simulink model "darkquad17"  (R2012b)
settings: Solver=VariableStepDiscrete  SolverMode=SingleTasking  StartTime=0.0  StopTime=10000  RelTol=1e-3
libraries: xbsIndex_r4 x6460, casper_library_misc x74, casper_library_flow_control x8, xps_library x7
(part 29 of 59)

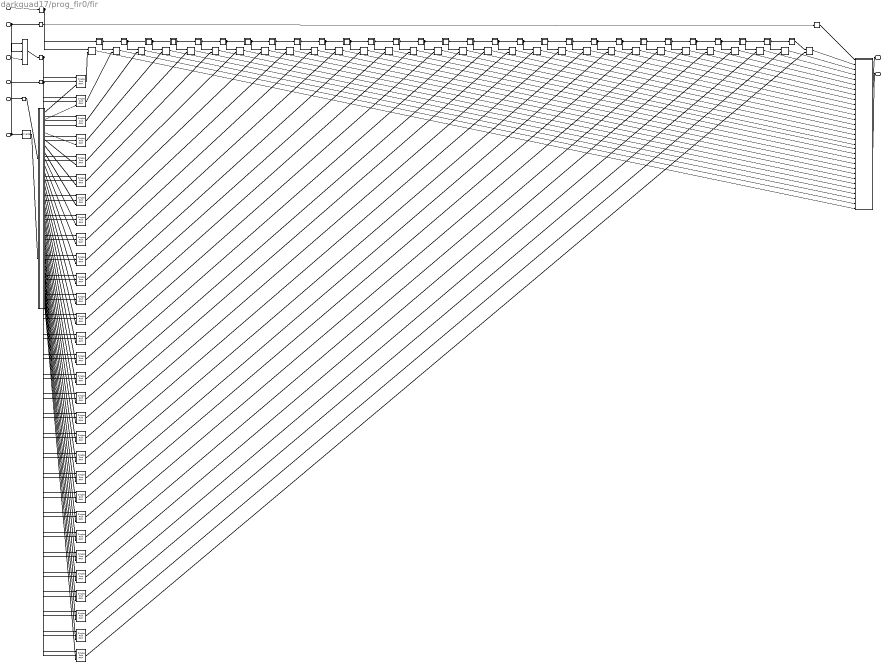
== system darkquad17/prog_fir0/fir ==
  data_in : Inport
  ch_in : Inport  Port=2
  write_coeff : Inport  Port=3
  coeff_to_write : Inport  Port=4
  tap_to_write : Inport  Port=5
  ch_to_write : Inport  Port=6
  Mult{1..30} (30 alike) : xbsIndex_r4/Mult  precision=Full  arith_type="Signed  (2's comp)"  n_bits=16  bin_pt=14  quantization=Truncate  overflow=Wrap  en=off  latency=4  dbl_ovrd=off  use_behavioral_HDL=off  opt=Speed  use_embedded=on  optimum_pipeline=on  pipeline=on  use_rpm=on  placement_style=Triangular  block_type=mult
  bram{1..30} (30 alike) : xbsIndex_r4/Single Port RAM  depth=256  initVector=0  distributed_mem=Block RAM  write_mode=No Read On Write  rst=off  init_reg=0  en=off  latency=3  dbl_ovrd=off  optimize=Area  block_type=spram
  ch_dly : xbsIndex_r4/Delay  rst=off  infoeditControl=Selection of Reset will increase slice count due to use of real FFs and instead of SRLs  en=off  latency=2  dbl_ovrd=off  reg_retiming=off  block_type=delay
  ch_mux : xbsIndex_r4/Mux  inputs=2  en=off  latency=1  precision=Full  arith_type=Unsigned  n_bits=16  bin_pt=14  quantization=Truncate  overflow=Wrap  dbl_ovrd=off  block_type=mux
  coeff_in_dly : xbsIndex_r4/Delay  rst=off  infoeditControl=Selection of Reset will increase slice count due to use of real FFs and instead of SRLs  en=off  latency=3  dbl_ovrd=off  reg_retiming=off  block_type=delay
  data_dly : xbsIndex_r4/Delay  rst=off  infoeditControl=Selection of Reset will increase slice count due to use of real FFs and instead of SRLs  en=off  latency=6  dbl_ovrd=off  reg_retiming=off  block_type=delay
  delay1 : Subsystem  mask(delay_bram){DelayLen=256, bram_latency=2, implementation=Fabric, async=off}
      mask prompts: DelayLen "Delay By:"; bram_latency "BRAM Latency"; implementation "Implement using"; async "asynchronous operation"
      mask help: A delay block that uses BRAM for its storage.
      mask init:
      | delay_bram_impl_init(gcb, ...
      |     'DelayLen', DelayLen, ...
      |     'bram_latency', bram_latency, ...
      |     'implementation', implementation, ...
      |     'async', async);
      mask Help: eval('xlWeb(''http://casper.berkeley.edu/wiki/Delay_bram'')')
      mask TypeOptions implementation: Behavioral HDL | Fabric | DSP48
      mask Display:
      | str=sprintf('z^{-%d}',DelayLen);
      | color('black');disp(str,'texmode','on');
  delay10 : Subsystem  mask(delay_bram){DelayLen=256, bram_latency=2, implementation=Fabric, async=off}
      mask prompts: DelayLen "Delay By:"; bram_latency "BRAM Latency"; implementation "Implement using"; async "asynchronous operation"
      mask help: A delay block that uses BRAM for its storage.
      mask init:
      | delay_bram_impl_init(gcb, ...
      |     'DelayLen', DelayLen, ...
      |     'bram_latency', bram_latency, ...
      |     'implementation', implementation, ...
      |     'async', async);
      mask Help: eval('xlWeb(''http://casper.berkeley.edu/wiki/Delay_bram'')')
      mask TypeOptions implementation: Behavioral HDL | Fabric | DSP48
      mask Display:
      | str=sprintf('z^{-%d}',DelayLen);
      | color('black');disp(str,'texmode','on');
  delay11 : Subsystem  mask(delay_bram){DelayLen=256, bram_latency=2, implementation=Fabric, async=off}
      mask prompts: DelayLen "Delay By:"; bram_latency "BRAM Latency"; implementation "Implement using"; async "asynchronous operation"
      mask help: A delay block that uses BRAM for its storage.
      mask init:
      | delay_bram_impl_init(gcb, ...
      |     'DelayLen', DelayLen, ...
      |     'bram_latency', bram_latency, ...
      |     'implementation', implementation, ...
      |     'async', async);
      mask Help: eval('xlWeb(''http://casper.berkeley.edu/wiki/Delay_bram'')')
      mask TypeOptions implementation: Behavioral HDL | Fabric | DSP48
      mask Display:
      | str=sprintf('z^{-%d}',DelayLen);
      | color('black');disp(str,'texmode','on');
  delay12 : Subsystem  mask(delay_bram){DelayLen=256, bram_latency=2, implementation=Fabric, async=off}
      mask prompts: DelayLen "Delay By:"; bram_latency "BRAM Latency"; implementation "Implement using"; async "asynchronous operation"
      mask help: A delay block that uses BRAM for its storage.
      mask init:
      | delay_bram_impl_init(gcb, ...
      |     'DelayLen', DelayLen, ...
      |     'bram_latency', bram_latency, ...
      |     'implementation', implementation, ...
      |     'async', async);
      mask Help: eval('xlWeb(''http://casper.berkeley.edu/wiki/Delay_bram'')')
      mask TypeOptions implementation: Behavioral HDL | Fabric | DSP48
      mask Display:
      | str=sprintf('z^{-%d}',DelayLen);
      | color('black');disp(str,'texmode','on');
  delay13 : Subsystem  mask(delay_bram){DelayLen=256, bram_latency=2, implementation=Fabric, async=off}
      mask prompts: DelayLen "Delay By:"; bram_latency "BRAM Latency"; implementation "Implement using"; async "asynchronous operation"
      mask help: A delay block that uses BRAM for its storage.
      mask init:
      | delay_bram_impl_init(gcb, ...
      |     'DelayLen', DelayLen, ...
      |     'bram_latency', bram_latency, ...
      |     'implementation', implementation, ...
      |     'async', async);
      mask Help: eval('xlWeb(''http://casper.berkeley.edu/wiki/Delay_bram'')')
      mask TypeOptions implementation: Behavioral HDL | Fabric | DSP48
      mask Display:
      | str=sprintf('z^{-%d}',DelayLen);
      | color('black');disp(str,'texmode','on');
  delay14 : Subsystem  mask(delay_bram){DelayLen=256, bram_latency=2, implementation=Fabric, async=off}
      mask prompts: DelayLen "Delay By:"; bram_latency "BRAM Latency"; implementation "Implement using"; async "asynchronous operation"
      mask help: A delay block that uses BRAM for its storage.
      mask init:
      | delay_bram_impl_init(gcb, ...
      |     'DelayLen', DelayLen, ...
      |     'bram_latency', bram_latency, ...
      |     'implementation', implementation, ...
      |     'async', async);
      mask Help: eval('xlWeb(''http://casper.berkeley.edu/wiki/Delay_bram'')')
      mask TypeOptions implementation: Behavioral HDL | Fabric | DSP48
      mask Display:
      | str=sprintf('z^{-%d}',DelayLen);
      | color('black');disp(str,'texmode','on');
  delay15 : Subsystem  mask(delay_bram){DelayLen=256, bram_latency=2, implementation=Fabric, async=off}
      mask prompts: DelayLen "Delay By:"; bram_latency "BRAM Latency"; implementation "Implement using"; async "asynchronous operation"
      mask help: A delay block that uses BRAM for its storage.
      mask init:
      | delay_bram_impl_init(gcb, ...
      |     'DelayLen', DelayLen, ...
      |     'bram_latency', bram_latency, ...
      |     'implementation', implementation, ...
      |     'async', async);
      mask Help: eval('xlWeb(''http://casper.berkeley.edu/wiki/Delay_bram'')')
      mask TypeOptions implementation: Behavioral HDL | Fabric | DSP48
      mask Display:
      | str=sprintf('z^{-%d}',DelayLen);
      | color('black');disp(str,'texmode','on');
  delay16 : Subsystem  mask(delay_bram){DelayLen=256, bram_latency=2, implementation=Fabric, async=off}
      mask prompts: DelayLen "Delay By:"; bram_latency "BRAM Latency"; implementation "Implement using"; async "asynchronous operation"
      mask help: A delay block that uses BRAM for its storage.
      mask init:
      | delay_bram_impl_init(gcb, ...
      |     'DelayLen', DelayLen, ...
      |     'bram_latency', bram_latency, ...
      |     'implementation', implementation, ...
      |     'async', async);
      mask Help: eval('xlWeb(''http://casper.berkeley.edu/wiki/Delay_bram'')')
      mask TypeOptions implementation: Behavioral HDL | Fabric | DSP48
      mask Display:
      | str=sprintf('z^{-%d}',DelayLen);
      | color('black');disp(str,'texmode','on');
  delay17 : Subsystem  mask(delay_bram){DelayLen=256, bram_latency=2, implementation=Fabric, async=off}
      mask prompts: DelayLen "Delay By:"; bram_latency "BRAM Latency"; implementation "Implement using"; async "asynchronous operation"
      mask help: A delay block that uses BRAM for its storage.
      mask init:
      | delay_bram_impl_init(gcb, ...
      |     'DelayLen', DelayLen, ...
      |     'bram_latency', bram_latency, ...
      |     'implementation', implementation, ...
      |     'async', async);
      mask Help: eval('xlWeb(''http://casper.berkeley.edu/wiki/Delay_bram'')')
      mask TypeOptions implementation: Behavioral HDL | Fabric | DSP48
      mask Display:
      | str=sprintf('z^{-%d}',DelayLen);
      | color('black');disp(str,'texmode','on');
  delay18 : Subsystem  mask(delay_bram){DelayLen=256, bram_latency=2, implementation=Fabric, async=off}
      mask prompts: DelayLen "Delay By:"; bram_latency "BRAM Latency"; implementation "Implement using"; async "asynchronous operation"
      mask help: A delay block that uses BRAM for its storage.
      mask init:
      | delay_bram_impl_init(gcb, ...
      |     'DelayLen', DelayLen, ...
      |     'bram_latency', bram_latency, ...
      |     'implementation', implementation, ...
      |     'async', async);
      mask Help: eval('xlWeb(''http://casper.berkeley.edu/wiki/Delay_bram'')')
      mask TypeOptions implementation: Behavioral HDL | Fabric | DSP48
      mask Display:
      | str=sprintf('z^{-%d}',DelayLen);
      | color('black');disp(str,'texmode','on');
  delay19 : Subsystem  mask(delay_bram){DelayLen=256, bram_latency=2, implementation=Fabric, async=off}
      mask prompts: DelayLen "Delay By:"; bram_latency "BRAM Latency"; implementation "Implement using"; async "asynchronous operation"
      mask help: A delay block that uses BRAM for its storage.
      mask init:
      | delay_bram_impl_init(gcb, ...
      |     'DelayLen', DelayLen, ...
      |     'bram_latency', bram_latency, ...
      |     'implementation', implementation, ...
      |     'async', async);
      mask Help: eval('xlWeb(''http://casper.berkeley.edu/wiki/Delay_bram'')')
      mask TypeOptions implementation: Behavioral HDL | Fabric | DSP48
      mask Display:
      | str=sprintf('z^{-%d}',DelayLen);
      | color('black');disp(str,'texmode','on');
  delay2 : Subsystem  mask(delay_bram){DelayLen=256, bram_latency=2, implementation=Fabric, async=off}
      mask prompts: DelayLen "Delay By:"; bram_latency "BRAM Latency"; implementation "Implement using"; async "asynchronous operation"
      mask help: A delay block that uses BRAM for its storage.
      mask init:
      | delay_bram_impl_init(gcb, ...
      |     'DelayLen', DelayLen, ...
      |     'bram_latency', bram_latency, ...
      |     'implementation', implementation, ...
      |     'async', async);
      mask Help: eval('xlWeb(''http://casper.berkeley.edu/wiki/Delay_bram'')')
      mask TypeOptions implementation: Behavioral HDL | Fabric | DSP48
      mask Display:
      | str=sprintf('z^{-%d}',DelayLen);
      | color('black');disp(str,'texmode','on');
  delay20 : Subsystem  mask(delay_bram){DelayLen=256, bram_latency=2, implementation=Fabric, async=off}
      mask prompts: DelayLen "Delay By:"; bram_latency "BRAM Latency"; implementation "Implement using"; async "asynchronous operation"
      mask help: A delay block that uses BRAM for its storage.
      mask init:
      | delay_bram_impl_init(gcb, ...
      |     'DelayLen', DelayLen, ...
      |     'bram_latency', bram_latency, ...
      |     'implementation', implementation, ...
      |     'async', async);
      mask Help: eval('xlWeb(''http://casper.berkeley.edu/wiki/Delay_bram'')')
      mask TypeOptions implementation: Behavioral HDL | Fabric | DSP48
      mask Display:
      | str=sprintf('z^{-%d}',DelayLen);
      | color('black');disp(str,'texmode','on');
  delay21 : Subsystem  mask(delay_bram){DelayLen=256, bram_latency=2, implementation=Fabric, async=off}
      mask prompts: DelayLen "Delay By:"; bram_latency "BRAM Latency"; implementation "Implement using"; async "asynchronous operation"
      mask help: A delay block that uses BRAM for its storage.
      mask init:
      | delay_bram_impl_init(gcb, ...
      |     'DelayLen', DelayLen, ...
      |     'bram_latency', bram_latency, ...
      |     'implementation', implementation, ...
      |     'async', async);
      mask Help: eval('xlWeb(''http://casper.berkeley.edu/wiki/Delay_bram'')')
      mask TypeOptions implementation: Behavioral HDL | Fabric | DSP48
      mask Display:
      | str=sprintf('z^{-%d}',DelayLen);
      | color('black');disp(str,'texmode','on');
  delay22 : Subsystem  mask(delay_bram){DelayLen=256, bram_latency=2, implementation=Fabric, async=off}
      mask prompts: DelayLen "Delay By:"; bram_latency "BRAM Latency"; implementation "Implement using"; async "asynchronous operation"
      mask help: A delay block that uses BRAM for its storage.
      mask init:
      | delay_bram_impl_init(gcb, ...
      |     'DelayLen', DelayLen, ...
      |     'bram_latency', bram_latency, ...
      |     'implementation', implementation, ...
      |     'async', async);
      mask Help: eval('xlWeb(''http://casper.berkeley.edu/wiki/Delay_bram'')')
      mask TypeOptions implementation: Behavioral HDL | Fabric | DSP48
      mask Display:
      | str=sprintf('z^{-%d}',DelayLen);
      | color('black');disp(str,'texmode','on');
  delay23 : Subsystem  mask(delay_bram){DelayLen=256, bram_latency=2, implementation=Fabric, async=off}
      mask prompts: DelayLen "Delay By:"; bram_latency "BRAM Latency"; implementation "Implement using"; async "asynchronous operation"
      mask help: A delay block that uses BRAM for its storage.
      mask init:
      | delay_bram_impl_init(gcb, ...
      |     'DelayLen', DelayLen, ...
      |     'bram_latency', bram_latency, ...
      |     'implementation', implementation, ...
      |     'async', async);
      mask Help: eval('xlWeb(''http://casper.berkeley.edu/wiki/Delay_bram'')')
      mask TypeOptions implementation: Behavioral HDL | Fabric | DSP48
      mask Display:
      | str=sprintf('z^{-%d}',DelayLen);
      | color('black');disp(str,'texmode','on');
  delay24 : Subsystem  mask(delay_bram){DelayLen=256, bram_latency=2, implementation=Fabric, async=off}
      mask prompts: DelayLen "Delay By:"; bram_latency "BRAM Latency"; implementation "Implement using"; async "asynchronous operation"
      mask help: A delay block that uses BRAM for its storage.
      mask init:
      | delay_bram_impl_init(gcb, ...
      |     'DelayLen', DelayLen, ...
      |     'bram_latency', bram_latency, ...
      |     'implementation', implementation, ...
      |     'async', async);
      mask Help: eval('xlWeb(''http://casper.berkeley.edu/wiki/Delay_bram'')')
      mask TypeOptions implementation: Behavioral HDL | Fabric | DSP48
      mask Display:
      | str=sprintf('z^{-%d}',DelayLen);
      | color('black');disp(str,'texmode','on');
  delay25 : Subsystem  mask(delay_bram){DelayLen=256, bram_latency=2, implementation=Fabric, async=off}
      mask prompts: DelayLen "Delay By:"; bram_latency "BRAM Latency"; implementation "Implement using"; async "asynchronous operation"
      mask help: A delay block that uses BRAM for its storage.
      mask init:
      | delay_bram_impl_init(gcb, ...
      |     'DelayLen', DelayLen, ...
      |     'bram_latency', bram_latency, ...
      |     'implementation', implementation, ...
      |     'async', async);
      mask Help: eval('xlWeb(''http://casper.berkeley.edu/wiki/Delay_bram'')')
      mask TypeOptions implementation: Behavioral HDL | Fabric | DSP48
      mask Display:
      | str=sprintf('z^{-%d}',DelayLen);
      | color('black');disp(str,'texmode','on');
  delay26 : Subsystem  mask(delay_bram){DelayLen=256, bram_latency=2, implementation=Fabric, async=off}
      mask prompts: DelayLen "Delay By:"; bram_latency "BRAM Latency"; implementation "Implement using"; async "asynchronous operation"
      mask help: A delay block that uses BRAM for its storage.
      mask init:
      | delay_bram_impl_init(gcb, ...
      |     'DelayLen', DelayLen, ...
      |     'bram_latency', bram_latency, ...
      |     'implementation', implementation, ...
      |     'async', async);
      mask Help: eval('xlWeb(''http://casper.berkeley.edu/wiki/Delay_bram'')')
      mask TypeOptions implementation: Behavioral HDL | Fabric | DSP48
      mask Display:
      | str=sprintf('z^{-%d}',DelayLen);
      | color('black');disp(str,'texmode','on');
  delay27 : Subsystem  mask(delay_bram){DelayLen=256, bram_latency=2, implementation=Fabric, async=off}
      mask prompts: DelayLen "Delay By:"; bram_latency "BRAM Latency"; implementation "Implement using"; async "asynchronous operation"
      mask help: A delay block that uses BRAM for its storage.
      mask init:
      | delay_bram_impl_init(gcb, ...
      |     'DelayLen', DelayLen, ...
      |     'bram_latency', bram_latency, ...
      |     'implementation', implementation, ...
      |     'async', async);
      mask Help: eval('xlWeb(''http://casper.berkeley.edu/wiki/Delay_bram'')')
      mask TypeOptions implementation: Behavioral HDL | Fabric | DSP48
      mask Display:
      | str=sprintf('z^{-%d}',DelayLen);
      | color('black');disp(str,'texmode','on');
  delay28 : Subsystem  mask(delay_bram){DelayLen=256, bram_latency=2, implementation=Fabric, async=off}
      mask prompts: DelayLen "Delay By:"; bram_latency "BRAM Latency"; implementation "Implement using"; async "asynchronous operation"
      mask help: A delay block that uses BRAM for its storage.
      mask init:
      | delay_bram_impl_init(gcb, ...
      |     'DelayLen', DelayLen, ...
      |     'bram_latency', bram_latency, ...
      |     'implementation', implementation, ...
      |     'async', async);
      mask Help: eval('xlWeb(''http://casper.berkeley.edu/wiki/Delay_bram'')')
      mask TypeOptions implementation: Behavioral HDL | Fabric | DSP48
      mask Display:
      | str=sprintf('z^{-%d}',DelayLen);
      | color('black');disp(str,'texmode','on');
  delay29 : Subsystem  mask(delay_bram){DelayLen=256, bram_latency=2, implementation=Fabric, async=off}
      mask prompts: DelayLen "Delay By:"; bram_latency "BRAM Latency"; implementation "Implement using"; async "asynchronous operation"
      mask help: A delay block that uses BRAM for its storage.
      mask init:
      | delay_bram_impl_init(gcb, ...
      |     'DelayLen', DelayLen, ...
      |     'bram_latency', bram_latency, ...
      |     'implementation', implementation, ...
      |     'async', async);
      mask Help: eval('xlWeb(''http://casper.berkeley.edu/wiki/Delay_bram'')')
      mask TypeOptions implementation: Behavioral HDL | Fabric | DSP48
      mask Display:
      | str=sprintf('z^{-%d}',DelayLen);
      | color('black');disp(str,'texmode','on');
  delay3 : Subsystem  mask(delay_bram){DelayLen=256, bram_latency=2, implementation=Fabric, async=off}
      mask prompts: DelayLen "Delay By:"; bram_latency "BRAM Latency"; implementation "Implement using"; async "asynchronous operation"
      mask help: A delay block that uses BRAM for its storage.
      mask init:
      | delay_bram_impl_init(gcb, ...
      |     'DelayLen', DelayLen, ...
      |     'bram_latency', bram_latency, ...
      |     'implementation', implementation, ...
      |     'async', async);
      mask Help: eval('xlWeb(''http://casper.berkeley.edu/wiki/Delay_bram'')')
      mask TypeOptions implementation: Behavioral HDL | Fabric | DSP48
      mask Display:
      | str=sprintf('z^{-%d}',DelayLen);
      | color('black');disp(str,'texmode','on');
  delay4 : Subsystem  mask(delay_bram){DelayLen=256, bram_latency=2, implementation=Fabric, async=off}
      mask prompts: DelayLen "Delay By:"; bram_latency "BRAM Latency"; implementation "Implement using"; async "asynchronous operation"
      mask help: A delay block that uses BRAM for its storage.
      mask init:
      | delay_bram_impl_init(gcb, ...
      |     'DelayLen', DelayLen, ...
      |     'bram_latency', bram_latency, ...
      |     'implementation', implementation, ...
      |     'async', async);
      mask Help: eval('xlWeb(''http://casper.berkeley.edu/wiki/Delay_bram'')')
      mask TypeOptions implementation: Behavioral HDL | Fabric | DSP48
      mask Display:
      | str=sprintf('z^{-%d}',DelayLen);
      | color('black');disp(str,'texmode','on');
  delay5 : Subsystem  mask(delay_bram){DelayLen=256, bram_latency=2, implementation=Fabric, async=off}
      mask prompts: DelayLen "Delay By:"; bram_latency "BRAM Latency"; implementation "Implement using"; async "asynchronous operation"
      mask help: A delay block that uses BRAM for its storage.
      mask init:
      | delay_bram_impl_init(gcb, ...
      |     'DelayLen', DelayLen, ...
      |     'bram_latency', bram_latency, ...
      |     'implementation', implementation, ...
      |     'async', async);
      mask Help: eval('xlWeb(''http://casper.berkeley.edu/wiki/Delay_bram'')')
      mask TypeOptions implementation: Behavioral HDL | Fabric | DSP48
      mask Display:
      | str=sprintf('z^{-%d}',DelayLen);
      | color('black');disp(str,'texmode','on');
  delay6 : Subsystem  mask(delay_bram){DelayLen=256, bram_latency=2, implementation=Fabric, async=off}
      mask prompts: DelayLen "Delay By:"; bram_latency "BRAM Latency"; implementation "Implement using"; async "asynchronous operation"
      mask help: A delay block that uses BRAM for its storage.
      mask init:
      | delay_bram_impl_init(gcb, ...
      |     'DelayLen', DelayLen, ...
      |     'bram_latency', bram_latency, ...
      |     'implementation', implementation, ...
      |     'async', async);
      mask Help: eval('xlWeb(''http://casper.berkeley.edu/wiki/Delay_bram'')')
      mask TypeOptions implementation: Behavioral HDL | Fabric | DSP48
      mask Display:
      | str=sprintf('z^{-%d}',DelayLen);
      | color('black');disp(str,'texmode','on');
  delay7 : Subsystem  mask(delay_bram){DelayLen=256, bram_latency=2, implementation=Fabric, async=off}
      mask prompts: DelayLen "Delay By:"; bram_latency "BRAM Latency"; implementation "Implement using"; async "asynchronous operation"
      mask help: A delay block that uses BRAM for its storage.
      mask init:
      | delay_bram_impl_init(gcb, ...
      |     'DelayLen', DelayLen, ...
      |     'bram_latency', bram_latency, ...
      |     'implementation', implementation, ...
      |     'async', async);
      mask Help: eval('xlWeb(''http://casper.berkeley.edu/wiki/Delay_bram'')')
      mask TypeOptions implementation: Behavioral HDL | Fabric | DSP48
      mask Display:
      | str=sprintf('z^{-%d}',DelayLen);
      | color('black');disp(str,'texmode','on');
  delay8 : Subsystem  mask(delay_bram){DelayLen=256, bram_latency=2, implementation=Fabric, async=off}
      mask prompts: DelayLen "Delay By:"; bram_latency "BRAM Latency"; implementation "Implement using"; async "asynchronous operation"
      mask help: A delay block that uses BRAM for its storage.
      mask init:
      | delay_bram_impl_init(gcb, ...
      |     'DelayLen', DelayLen, ...
      |     'bram_latency', bram_latency, ...
      |     'implementation', implementation, ...
      |     'async', async);
      mask Help: eval('xlWeb(''http://casper.berkeley.edu/wiki/Delay_bram'')')
      mask TypeOptions implementation: Behavioral HDL | Fabric | DSP48
      mask Display:
      | str=sprintf('z^{-%d}',DelayLen);
      | color('black');disp(str,'texmode','on');
  delay9 : Subsystem  mask(delay_bram){DelayLen=256, bram_latency=2, implementation=Fabric, async=off}
      mask prompts: DelayLen "Delay By:"; bram_latency "BRAM Latency"; implementation "Implement using"; async "asynchronous operation"
      mask help: A delay block that uses BRAM for its storage.
      mask init:
      | delay_bram_impl_init(gcb, ...
      |     'DelayLen', DelayLen, ...
      |     'bram_latency', bram_latency, ...
      |     'implementation', implementation, ...
      |     'async', async);
      mask Help: eval('xlWeb(''http://casper.berkeley.edu/wiki/Delay_bram'')')
      mask TypeOptions implementation: Behavioral HDL | Fabric | DSP48
      mask Display:
      | str=sprintf('z^{-%d}',DelayLen);
      | color('black');disp(str,'texmode','on');
  demux : Subsystem  mask(demux){nOutputs=30, provideEnable=on}
      mask prompts: nOutputs "number of outputs"; provideEnable "provide enable port"
      mask init:
      | demux_init(gcb,'nOutputs',nOutputs,'provideEnable',provideEnable);
  misc_dly : xbsIndex_r4/Delay  rst=off  infoeditControl=Selection of Reset will increase slice count due to use of real FFs and instead of SRLs  en=off  latency=6  dbl_ovrd=off  reg_retiming=off  block_type=delay
  not_clear : xbsIndex_r4/Inverter  en=off  latency=1  dbl_ovrd=off  block_type=inv
  sum : Subsystem  AncestorBlock=casper_library_misc/adder_tree  mask(adder_tree){n_inputs=30, latency=3, adder_imp=DSP48, first_stage_hdl=on}
      mask prompts: n_inputs "Number of Inputs"; latency "Add Latency"; adder_imp "Adder implementation"; first_stage_hdl "Use behavioural HDL for first stage of adders"
      mask help:
      | Sums all inputs using a tree of adds and delays.
      |
      | Number of inputs: The number of inputs to the block to be summed
      | Add latency: The number of clock cycles to perform one addition (affects timing)..
      | Adder implementation: choice of fabric or DSP48E core, or behavioral HDL
      | Use behavioural HDL for first stage of adders: Causes the first stage of adders to be absorbed into DSP blocks if multipliers precede them (Virtex 5). Overrides Adder implementation
      mask init:
      | adder_tree_init(gcb, ...
      |     'n_inputs', n_inputs, ...
      |     'latency', latency, ...
      |     'adder_imp', adder_imp, ...
      |     'first_stage_hdl', first_stage_hdl);
      settings: AttributesFormatString=latency 15
      mask Help: eval('xlWeb(''http://casper.berkeley.edu/wiki/Adder_tree'')')
      mask TypeOptions adder_imp: Behavioral | Fabric | DSP48
  sync_delay : xbsIndex_r4/Delay  rst=off  infoeditControl=Selection of Reset will increase slice count due to use of real FFs and instead of SRLs  en=off  latency=4  dbl_ovrd=off  reg_retiming=off  block_type=delay
  tap_dly : xbsIndex_r4/Delay  rst=off  infoeditControl=Selection of Reset will increase slice count due to use of real FFs and instead of SRLs  en=off  latency=1  dbl_ovrd=off  reg_retiming=off  block_type=delay
  data_out : Outport
  ch_out : Outport  Port=2
  wires:
  ch_in/1 -> misc_dly/1, ch_mux/2
  ch_to_write/1 -> ch_mux/3
  write_coeff/1 -> ch_mux/1, not_clear/1
  ch_mux/1 -> ch_dly/1
  tap_to_write/1 -> tap_dly/1
  coeff_to_write/1 -> coeff_in_dly/1
  misc_dly/1 -> sync_delay/1
  sum/2(dout) -> data_out/1
  sync_delay/1 -> sum/1(sync)
  sum/1(sync_out) -> ch_out/1
  tap_dly/1 -> demux/1(in)
  not_clear/1 -> demux/2(clear)
  Mult1/1 -> sum/31(din30)
  bram1/1 -> Mult1/2
  ch_dly/1 -> bram1/1, bram2/1, bram3/1, bram4/1, bram5/1, bram6/1, bram7/1, bram8/1, bram9/1, bram10/1, bram11/1, bram12/1, bram13/1, bram14/1, bram15/1, bram16/1, bram17/1, bram18/1, bram19/1, bram20/1, bram21/1, bram22/1, bram23/1, bram24/1, bram25/1, bram26/1, bram27/1, bram28/1, bram29/1, bram30/1
  coeff_in_dly/1 -> bram1/2, bram2/2, bram3/2, bram4/2, bram5/2, bram6/2, bram7/2, bram8/2, bram9/2, bram10/2, bram11/2, bram12/2, bram13/2, bram14/2, bram15/2, bram16/2, bram17/2, bram18/2, bram19/2, bram20/2, bram21/2, bram22/2, bram23/2, bram24/2, bram25/2, bram26/2, bram27/2, bram28/2, bram29/2, bram30/2
  demux/1(out0) -> bram1/3
  delay1/1(dout) -> Mult2/1, delay2/1(din)
  Mult2/1 -> sum/30(din29)
  bram2/1 -> Mult2/2
  demux/2(out1) -> bram2/3
  delay2/1(dout) -> Mult3/1, delay3/1(din)
  Mult3/1 -> sum/29(din28)
  bram3/1 -> Mult3/2
  demux/3(out2) -> bram3/3
  delay3/1(dout) -> Mult4/1, delay4/1(din)
  Mult4/1 -> sum/28(din27)
  bram4/1 -> Mult4/2
  demux/4(out3) -> bram4/3
  delay4/1(dout) -> Mult5/1, delay5/1(din)
  Mult5/1 -> sum/27(din26)
  bram5/1 -> Mult5/2
  demux/5(out4) -> bram5/3
  delay5/1(dout) -> Mult6/1, delay6/1(din)
  Mult6/1 -> sum/26(din25)
  bram6/1 -> Mult6/2
  demux/6(out5) -> bram6/3
  delay6/1(dout) -> Mult7/1, delay7/1(din)
  Mult7/1 -> sum/25(din24)
  bram7/1 -> Mult7/2
  demux/7(out6) -> bram7/3
  delay7/1(dout) -> Mult8/1, delay8/1(din)
  Mult8/1 -> sum/24(din23)
  bram8/1 -> Mult8/2
  demux/8(out7) -> bram8/3
  delay8/1(dout) -> Mult9/1, delay9/1(din)
  Mult9/1 -> sum/23(din22)
  bram9/1 -> Mult9/2
  demux/9(out8) -> bram9/3
  delay9/1(dout) -> Mult10/1, delay10/1(din)
  Mult10/1 -> sum/22(din21)
  bram10/1 -> Mult10/2
  demux/10(out9) -> bram10/3
  delay10/1(dout) -> Mult11/1, delay11/1(din)
  Mult11/1 -> sum/21(din20)
  bram11/1 -> Mult11/2
  demux/11(out10) -> bram11/3
  delay11/1(dout) -> Mult12/1, delay12/1(din)
  Mult12/1 -> sum/20(din19)
  bram12/1 -> Mult12/2
  demux/12(out11) -> bram12/3
  delay12/1(dout) -> Mult13/1, delay13/1(din)
  Mult13/1 -> sum/19(din18)
  bram13/1 -> Mult13/2
  demux/13(out12) -> bram13/3
  delay13/1(dout) -> Mult14/1, delay14/1(din)
  Mult14/1 -> sum/18(din17)
  bram14/1 -> Mult14/2
  demux/14(out13) -> bram14/3
  delay14/1(dout) -> Mult15/1, delay15/1(din)
  Mult15/1 -> sum/17(din16)
  bram15/1 -> Mult15/2
  demux/15(out14) -> bram15/3
  delay15/1(dout) -> Mult16/1, delay16/1(din)
  Mult16/1 -> sum/16(din15)
  bram16/1 -> Mult16/2
  demux/16(out15) -> bram16/3
  delay16/1(dout) -> Mult17/1, delay17/1(din)
  Mult17/1 -> sum/15(din14)
  bram17/1 -> Mult17/2
  demux/17(out16) -> bram17/3
  delay17/1(dout) -> Mult18/1, delay18/1(din)
  Mult18/1 -> sum/14(din13)
  bram18/1 -> Mult18/2
  demux/18(out17) -> bram18/3
  delay18/1(dout) -> Mult19/1, delay19/1(din)
  Mult19/1 -> sum/13(din12)
  bram19/1 -> Mult19/2
  demux/19(out18) -> bram19/3
  delay19/1(dout) -> Mult20/1, delay20/1(din)
  Mult20/1 -> sum/12(din11)
  bram20/1 -> Mult20/2
  demux/20(out19) -> bram20/3
  delay20/1(dout) -> Mult21/1, delay21/1(din)
  Mult21/1 -> sum/11(din10)
  bram21/1 -> Mult21/2
  demux/21(out20) -> bram21/3
  delay21/1(dout) -> Mult22/1, delay22/1(din)
  Mult22/1 -> sum/10(din9)
  bram22/1 -> Mult22/2
  demux/22(out21) -> bram22/3
  delay22/1(dout) -> Mult23/1, delay23/1(din)
  Mult23/1 -> sum/9(din8)
  bram23/1 -> Mult23/2
  demux/23(out22) -> bram23/3
  delay23/1(dout) -> Mult24/1, delay24/1(din)
  Mult24/1 -> sum/8(din7)
  bram24/1 -> Mult24/2
  demux/24(out23) -> bram24/3
  delay24/1(dout) -> Mult25/1, delay25/1(din)
  Mult25/1 -> sum/7(din6)
  bram25/1 -> Mult25/2
  demux/25(out24) -> bram25/3
  delay25/1(dout) -> Mult26/1, delay26/1(din)
  Mult26/1 -> sum/6(din5)
  bram26/1 -> Mult26/2
  demux/26(out25) -> bram26/3
  delay26/1(dout) -> Mult27/1, delay27/1(din)
  Mult27/1 -> sum/5(din4)
  bram27/1 -> Mult27/2
  demux/27(out26) -> bram27/3
  delay27/1(dout) -> Mult28/1, delay28/1(din)
  Mult28/1 -> sum/4(din3)
  bram28/1 -> Mult28/2
  demux/28(out27) -> bram28/3
  delay28/1(dout) -> Mult29/1, delay29/1(din)
  Mult29/1 -> sum/3(din2)
  bram29/1 -> Mult29/2
  demux/29(out28) -> bram29/3
  delay29/1(dout) -> Mult30/1
  Mult30/1 -> sum/2(din1)
  bram30/1 -> Mult30/2
  demux/30(out29) -> bram30/3
  data_in/1 -> data_dly/1
  data_dly/1 -> delay1/1(din), Mult1/1

== system darkquad17/prog_fir0/load_chan ==
  darkquad17_prog_fir0_load_chan_user_data_out : xbsIndex_r4/Gateway In  gui_display_data_type=Fixed-point  arith_type=Unsigned  n_bits=32  bin_pt=0  preci_type=Single  exp_width=8  frac_width=24  quantization="Round  (unbiased: +/- Inf)"  overflow=Saturate  period=1  dbl_ovrd=off  timing_constraint=None  locs_specified=off  LOCs={}  UseAsADC=off  ADCChannel='1'  inherit_from_input=off  hdl_port=on  block_type=gatewayin
  io_delay : xbsIndex_r4/Delay  rst=off  infoeditControl=Selection of Reset will increase slice count due to use of real FFs and instead of SRLs  en=off  latency=0  dbl_ovrd=off  reg_retiming=on  block_type=delay
  reint1 : xbsIndex_r4/Reinterpret  force_arith_type=on  arith_type=Unsigned  force_bin_pt=on  bin_pt=0  block_type=reinterpret
  sim_1 : Constant  Value=0
  slice_reg : xbsIndex_r4/Slice  nbits=32  boolean_output=off  mode=Lower Bit Location + Width  bit1=0  base1=MSB of Input  bit0=0  base0=LSB of Input  dbl_ovrd=off  block_type=slice
  in_reg : Outport
  wires:
  darkquad17_prog_fir0_load_chan_user_data_out/1 -> io_delay/1
  sim_1/1 -> darkquad17_prog_fir0_load_chan_user_data_out/1
  io_delay/1 -> slice_reg/1
  slice_reg/1 -> reint1/1
  reint1/1 -> in_reg/1

== system darkquad17/prog_fir0/pipeline1 ==
  d : Inport
  Register0 : xbsIndex_r4/Register  init=0  rst=off  en=off  dbl_ovrd=off  block_type=register
      settings: block_version=11.4
  Register1 : xbsIndex_r4/Register  init=0  rst=off  en=off  dbl_ovrd=off  block_type=register
      settings: block_version=11.4
  q : Outport
  wires:
  Register0/1 -> Register1/1
  d/1 -> Register0/1
  Register1/1 -> q/1

== system darkquad17/prog_fir0/single_chan_coeffs ==
  addr : Inport
  data_in : Inport  Port=2
  we : Inport  Port=3
  calc_add : Subsystem  mask{data_width=32, addr_width=10, sample_rate=sample_rate}
      mask prompts: data_width "data width"; addr_width "address width"; sample_rate "sample rate"
  convert_addr : xbsIndex_r4/Convert  gui_display_data_type=Fixed-point  arith_type=Unsigned  n_bits=addr_width  bin_pt=0  float_type=Single  exp_bits=8  fraction_bits=24  quantization=Truncate  overflow=Wrap  en=off  latency=0  dbl_ovrd=off  pipeline=off  block_type=convert
      settings: xl_area=[0, 0, 0, 0, 0, 0, 0]
  convert_din1 : xbsIndex_r4/Convert  gui_display_data_type=Fixed-point  arith_type=Unsigned  n_bits=32  bin_pt=0  float_type=Single  exp_bits=8  fraction_bits=24  quantization=Truncate  overflow=Wrap  en=off  latency=0  dbl_ovrd=off  pipeline=off  block_type=convert
      settings: xl_area=[0, 0, 0, 0, 0, 0, 0]
  convert_we : xbsIndex_r4/Convert  gui_display_data_type=Fixed-point  arith_type=Unsigned  n_bits=1  bin_pt=0  float_type=Single  exp_bits=8  fraction_bits=24  quantization=Truncate  overflow=Wrap  en=off  latency=0  dbl_ovrd=off  pipeline=off  block_type=convert
      settings: xl_area=[0, 0, 0, 0, 0, 0, 0]
  darkquad17_prog_fir0_single_chan_coeffs_addr : xbsIndex_r4/Gateway Out  inherit_from_input=off  hdl_port=on  timing_constraint=None  locs_specified=off  LOCs={'A5','B9','A9','C1','A3','G6','E9','A6','A7','A8','B8','B1','B3','D9','B5','B4','B6','C2'}  UseAsDAC=off  DACChannel='1'  block_type=gatewayout
      settings: infoedit="Gateway out block.  Converts Xilinx fixed point inputs into ouputs of type Simulink integer, double, or fixed point.<P><P>Hardware notes:  In hardware these blocks become top level output ports or are discarded, depending on how they are configured."  xl_area=[0, 0, 0, 0, 0, 0, 0]  sginterface={'Nallatech'=>{'xdspkit'=>{'non_memory_mapped_port'=>'uprev_Shared_BRAM_addr'}},'Xilinx'=>{'jtaghwcosim'=>{'non_memory_mapped_port'=>'uprev_Shared_BRAM_addr'},'xdspkit'=>{'non_memory_mapped_port'=>'uprev_Shared_BRAM_addr'}}}
  darkquad17_prog_fir0_single_chan_coeffs_data_in : xbsIndex_r4/Gateway Out  inherit_from_input=off  hdl_port=on  timing_constraint=None  locs_specified=off  LOCs={'B21','B22','A22','B23','B19','C19','A20','A21','A23','B24','A24','A25','E18','D18','C18','B18'}  UseAsDAC=off  DACChannel='1'  block_type=gatewayout
      settings: infoedit="Gateway out block.  Converts Xilinx fixed point inputs into ouputs of type Simulink integer, double, or fixed point.<P><P>Hardware notes:  In hardware these blocks become top level output ports or are discarded, depending on how they are configured."  xl_area=[0, 0, 0, 0, 0, 0, 0]  sginterface={'Nallatech'=>{'xdspkit'=>{'non_memory_mapped_port'=>'uprev_Shared_BRAM_data_in'}},'Xilinx'=>{'jtaghwcosim'=>{'non_memory_mapped_port'=>'uprev_Shared_BRAM_data_in'},'xdspkit'=>{'non_memory_mapped_port'=>'uprev_Shared_BRAM_data_in'}}}
  darkquad17_prog_fir0_single_chan_coeffs_data_out : xbsIndex_r4/Gateway In  gui_display_data_type=Fixed-point  arith_type=Unsigned  n_bits=32  bin_pt=0  preci_type=Single  exp_width=8  frac_width=24  quantization=Truncate  overflow=Wrap  period=sample_rate  dbl_ovrd=off  timing_constraint=None  locs_specified=off  LOCs={}  UseAsADC=off  ADCChannel='1'  inherit_from_input=off  hdl_port=on  block_type=gatewayin
      settings: xl_area=[0, 0, 0, 0, 0, 0, 0]
  darkquad17_prog_fir0_single_chan_coeffs_we : xbsIndex_r4/Gateway Out  inherit_from_input=off  hdl_port=on  timing_constraint=None  locs_specified=off  LOCs={'A14'}  UseAsDAC=off  DACChannel='1'  block_type=gatewayout
      settings: infoedit="Gateway out block.  Converts Xilinx fixed point inputs into ouputs of type Simulink integer, double, or fixed point.<P><P>Hardware notes:  In hardware these blocks become top level output ports or are discarded, depending on how they are configured."  xl_area=[0, 0, 0, 0, 0, 0, 0]
  mem : Subsystem
  munge_in : Subsystem  AncestorBlock=casper_library_flow_control/munge  mask(munge){divisions=1, div_size=32, order=[0], arith_type_out=Unsigned, bin_pt_out=0}
      mask prompts: divisions "Number of divisions"; div_size "Division size (bits)"; order "Division packing order"; arith_type_out "Output arithmetic type"; bin_pt_out "Output binary point"
      mask help: Splits an input bus into the specified number of divisions and then recombines them in the order specified (most significant division = 0,least = number divisions-1)
      mask init:
      | munge_init(gcb, ...
      |     'divisions', divisions, ...
      |     'div_size', div_size, ...
      |     'order', order, ...
      |     'arith_type_out', arith_type_out, ...
      |     'bin_pt_out', bin_pt_out);
      settings: AttributesFormatString=|
      | split:32
      | join:0
      | Unsigned [32,0]
      mask TypeOptions arith_type_out: Unsigned | Signed  (2's comp) | Floating-point
  munge_out : Subsystem  AncestorBlock=casper_library_flow_control/munge  mask(munge){divisions=1, div_size=32, order=[0], arith_type_out=Unsigned, bin_pt_out=0}
      mask prompts: divisions "Number of divisions"; div_size "Division size (bits)"; order "Division packing order"; arith_type_out "Output arithmetic type"; bin_pt_out "Output binary point"
      mask help: Splits an input bus into the specified number of divisions and then recombines them in the order specified (most significant division = 0,least = number divisions-1)
      mask init:
      | munge_init(gcb, ...
      |     'divisions', divisions, ...
      |     'div_size', div_size, ...
      |     'order', order, ...
      |     'arith_type_out', arith_type_out, ...
      |     'bin_pt_out', bin_pt_out);
      settings: AttributesFormatString=|
      | split:32
      | join:0
      | Unsigned [32,0]
      mask TypeOptions arith_type_out: Unsigned | Signed  (2's comp) | Floating-point
  data_out : Outport
  wires:
  convert_addr/1 -> darkquad17_prog_fir0_single_chan_coeffs_addr/1
  convert_din1/1 -> darkquad17_prog_fir0_single_chan_coeffs_data_in/1
  data_in/1 -> munge_in/1(din)
  calc_add/1(out) -> convert_addr/1
  darkquad17_prog_fir0_single_chan_coeffs_we/1 -> mem/3(In3)
  darkquad17_prog_fir0_single_chan_coeffs_data_in/1 -> mem/2(In2)
  darkquad17_prog_fir0_single_chan_coeffs_addr/1 -> mem/1(In1)
  convert_we/1 -> darkquad17_prog_fir0_single_chan_coeffs_we/1
  darkquad17_prog_fir0_single_chan_coeffs_data_out/1 -> munge_out/1(din)
  mem/1(Out1) -> darkquad17_prog_fir0_single_chan_coeffs_data_out/1
  addr/1 -> calc_add/1(in)
  we/1 -> convert_we/1
  munge_out/1(dout) -> data_out/1
  munge_in/1(dout) -> convert_din1/1

== system darkquad17/prog_fir1/bus_expand2 ==
  bus_in : Inport
  reinterpret1 : xbsIndex_r4/Reinterpret  force_arith_type=on  arith_type=Unsigned  force_bin_pt=on  bin_pt=0  block_type=reinterpret
  reinterpret3 : xbsIndex_r4/Reinterpret  force_arith_type=on  arith_type=Unsigned  force_bin_pt=on  bin_pt=0  block_type=reinterpret
  slice1 : xbsIndex_r4/Slice  nbits=8  boolean_output=off  mode=Upper Bit Location + Width  bit1=-24  base1=MSB of Input  bit0=0  base0=LSB of Input  dbl_ovrd=off  block_type=slice
  slice2 : xbsIndex_r4/Slice  nbits=1  boolean_output=on  mode=Upper Bit Location + Width  bit1=-23  base1=MSB of Input  bit0=0  base0=LSB of Input  dbl_ovrd=off  block_type=slice
  slice3 : xbsIndex_r4/Slice  nbits=23  boolean_output=off  mode=Upper Bit Location + Width  bit1=0  base1=MSB of Input  bit0=0  base0=LSB of Input  dbl_ovrd=off  block_type=slice
  msb_out3 : Outport
  out2 : Outport  Port=2
  lsb_out1 : Outport  Port=3
  wires:
  reinterpret1/1 -> lsb_out1/1
  slice1/1 -> reinterpret1/1
  slice2/1 -> out2/1
  reinterpret3/1 -> msb_out3/1
  slice3/1 -> reinterpret3/1
  bus_in/1 -> slice1/1, slice2/1, slice3/1
